simulink subsystem "force_sensor"  (R2023b)
settings: Solver=VariableStepAuto  StartTime=0.0  StopTime=10.0  RelTol=1e-3
model mask{Ts=0.001}
  mask prompts: Ts "Sampling Time"
libraries: mbedblockslib x1
settings Model: Creator=kiraa  LastModifiedBy=kiraa

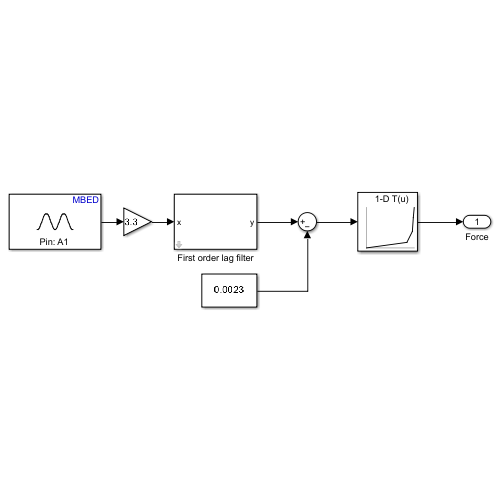
[thumbnail: Simulink's stored preview of the top-level diagram]
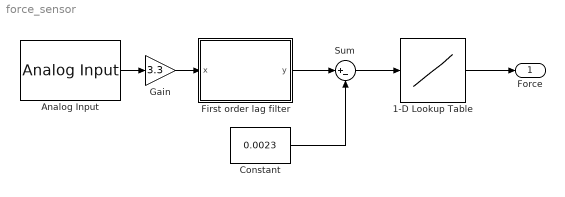
== system force_sensor ==
  1-D Lookup Table : Lookup_n-D  NumberOfTableDimensions=1  BreakpointsForDimension1=[0 2.605 3.003 3.053 3.087]  Table=[0 0.101 0.302 0.552 0.737]  InternalRulePriority=Speed  RndMeth=Simplest
  Analog Input : mbedblockslib/Analog Input  Pin=A1  ReadResultsOnly=off  ConversionTriggerSource=Software  ExternalTriggerType=uint32( 0 )  OutputDataType=double  EnableConversionCompleteNotify=off  EnableOuputStatus=off  SampleTime=Ts
      settings: LibrarySourceBlock=stmnucleorootlib/Common/Analog Input
  Constant : Constant  Value=0.0023
  First order lag filter : Subsystem  mask{Ts=0.001, alpha=exp(-0.001*20)}
      mask prompts: Ts "Filter sampling period"
  Gain : Gain  Gain=3.3
  Sum : Sum  Inputs=|+-
  Force : Outport
  wires:
  Analog Input/1 -> Gain/1
  1-D Lookup Table/1 -> Force/1
  Gain/1 -> First order lag filter/1(x)
  First order lag filter/1(y) -> Sum/1
  Constant/1 -> Sum/2
  Sum/1 -> 1-D Lookup Table/1

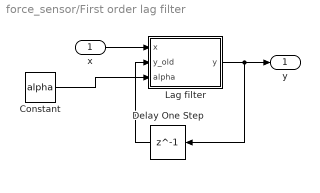
== system force_sensor/First order lag filter ==
  x : Inport
  Constant : Constant  Value=alpha
  Delay One Step : Delay  DelayLength=1  SampleTime=Ts
  Lag filter : MATLAB Function  TreatAsAtomicUnit=on
  y : Outport
  wires:
  Lag filter/1(y) -> y/1, Delay One Step/1
  Delay One Step/1 -> Lag filter/2(y_old)
  x/1 -> Lag filter/1(x)
  Constant/1 -> Lag filter/3(alpha)

== matlab function force_sensor/First order lag filter/Lag filter ==
  data: x input; y output; y_old input; alpha input
function y = fcn(x, y_old, alpha)
y = alpha*y_old+(1-alpha)*x;
